simulink model "cpu_sim"  (R2025b)
settings: Solver=VariableStepAuto  StartTime=0.0  StopTime=100  RelTol=1e-3
libraries: simulink x19, hdlsllib x7, embmathops x1
settings Model: Creator=karbi  LastModifiedBy=karbi

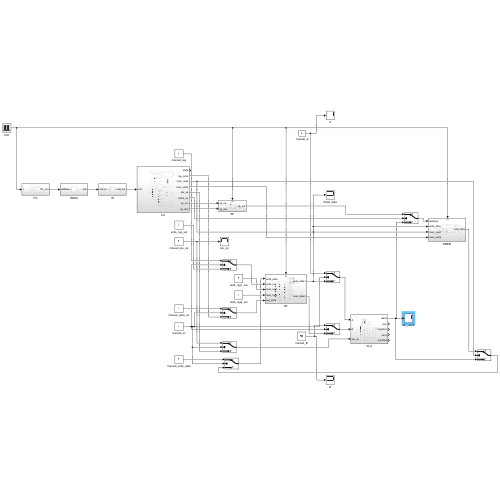
[thumbnail: Simulink's stored preview of the top-level diagram]
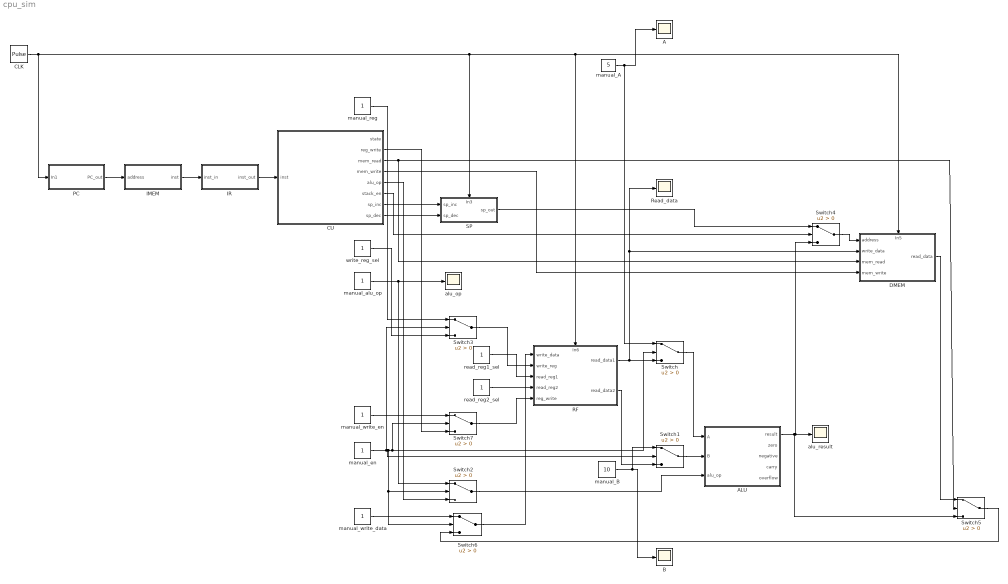
== system cpu_sim ==
  A : Scope
  ALU : Subsystem
  B : Scope
      settings: ActiveDisplayYMinimum=0.50000000000000011  ActiveDisplayYMaximum=5.5
  CLK : DiscretePulseGenerator  PulseType=Time based  Period=10  PulseWidth=5
  CU : Subsystem
  DMEM : Subsystem
      settings: PortSchema="{\"entries\":[{\"content\":{\"sides\":[{\"content\":{\"connectorIds\":[\"In1\",\"In2\",\"In3\",\"In4\"]},\"type\":\"ConnectorPlacement.EquallySpacedRectSide\",\"uuid\":\"c20ba0b8-e86b-4c3c-b1e7-27bfbe6d7ace\"},{\"content\":{\"connectorIds\":[\"Out1\"],\"side\":\"RIGHT\"},\"type\":\"ConnectorPlacement.EquallySpacedRectSide\",\"uuid\":\"6dfc7f35-ab74-4cab-b190-60f3ce7867eb\"},{\"content\":{\"connectorIds\":[\"In5\"],\"side\":\"TOP\"},\"type\":\"ConnectorPlacement.EquallySpacedRectSide\",\"uuid\":\"6a617f88-98bd-4419-a501-824654a091cc\"}]},\"type\":\"ConnectorPlacement.EquallySpacedConnector\",\"uuid\":\"d46b2777-b6fa-41c3-b118-b623252993db\"}],\"packageUris\":[\"http://schema.mathworks.com/mf0/Connector/R2020b\"],\"version\":\"1.0\"}"
  IMEM : Subsystem
  IR : Subsystem
  PC : Subsystem
  RF : Subsystem
      settings: PortSchema="{\"entries\":[{\"content\":{\"sides\":[{\"content\":{\"connectorIds\":[\"In1\",\"In2\",\"In3\",\"In4\",\"In5\"]},\"type\":\"ConnectorPlacement.EquallySpacedRectSide\",\"uuid\":\"b2b0e2f7-f1bc-4913-8ebd-763bbe465d15\"},{\"content\":{\"connectorIds\":[\"Out1\",\"Out2\"],\"side\":\"RIGHT\"},\"type\":\"ConnectorPlacement.EquallySpacedRectSide\",\"uuid\":\"2e2cea93-7dcf-43f8-b2d4-b46fbcb89eb4\"},{\"content\":{\"connectorIds\":[\"In6\"],\"side\":\"TOP\"},\"type\":\"ConnectorPlacement.EquallySpacedRectSide\",\"uuid\":\"73c40681-d123-4d1e-a253-0478733a22e7\"}]},\"type\":\"ConnectorPlacement.EquallySpacedConnector\",\"uuid\":\"66946b18-2392-495c-9280-4c233a61f8fd\"}],\"packageUris\":[\"http://schema.mathworks.com/mf0/Connector/R2020b\"],\"version\":\"1.0\"}"
  Read_data : Scope
      settings: DataLoggingVariableName=ScopeData3
  SP : Subsystem
      settings: PortSchema="{\"entries\":[{\"content\":{\"sides\":[{\"content\":{\"connectorIds\":[\"In1\",\"In2\"]},\"type\":\"ConnectorPlacement.EquallySpacedRectSide\",\"uuid\":\"dbfb5c57-0778-4d2f-89d9-125f1cc5ff40\"},{\"content\":{\"connectorIds\":[\"Out1\"],\"side\":\"RIGHT\"},\"type\":\"ConnectorPlacement.EquallySpacedRectSide\",\"uuid\":\"49ad81b3-cdaa-431a-a3c2-5d84586127d8\"},{\"content\":{\"connectorIds\":[\"In3\"],\"side\":\"TOP\"},\"type\":\"ConnectorPlacement.EquallySpacedRectSide\",\"uuid\":\"61861e8f-55bc-4e95-b317-e383488d79d7\"}]},\"type\":\"ConnectorPlacement.EquallySpacedConnector\",\"uuid\":\"436b8ade-eba4-422b-8f20-150aeb943b61\"}],\"packageUris\":[\"http://schema.mathworks.com/mf0/Connector/R2020b\"],\"version\":\"1.0\"}"
  Switch{,1..7} (8 alike) : Switch  Criteria=u2 > Threshold  SaturateOnIntegerOverflow=off  InputSameDT=off
  alu_op : Scope
      settings: DataLoggingVariableName=ScopeData2
  alu_result : Scope
      settings: ActiveDisplayYMinimum=-0.12200920583340213  ActiveDisplayYMaximum=10.004635007877717  DataLoggingVariableName=ScopeData4
  manual_A : Constant  Value=5  OutDataTypeStr=uint8
  manual_B : Constant  Value=10  OutDataTypeStr=uint8
  manual_alu_op : Constant  OutDataTypeStr=uint8
  manual_en : Constant  OutDataTypeStr=boolean
  manual_reg : Constant  OutDataTypeStr=uint8
  manual_write_data : Constant  OutDataTypeStr=uint8
  manual_write_en : Constant  OutDataTypeStr=boolean
  read_reg1_sel : Constant  OutDataTypeStr=uint8
  read_reg2_sel : Constant  OutDataTypeStr=uint8
  write_reg_sel : Constant  OutDataTypeStr=uint8
  wires:
  CU/4(mem_write) -> DMEM/4(mem_write)
  CU/3(mem_read) -> DMEM/3(mem_read), Switch5/2
  CU/2(reg_write) -> Switch7/3
  CU/6(stack_en) -> Switch4/2
  CLK/1 -> DMEM/5(In5), RF/6(In6), SP/3(In3), PC/1(In1)
  IR/1(inst_out) -> CU/1(inst)
  PC/1(PC_out) -> IMEM/1(address)
  IMEM/1(inst) -> IR/1(inst_in)
  manual_reg/1 -> Switch3/1
  CU/5(alu_op) -> Switch2/3
  CU/7(sp_inc) -> SP/1(sp_inc)
  CU/8(sp_dec) -> SP/2(sp_dec)
  manual_B/1 -> B/1, Switch1/1
  write_reg_sel/1 -> Switch3/3
  manual_alu_op/1 -> Switch2/1, alu_op/1
  manual_write_en/1 -> Switch7/1
  manual_en/1 -> Switch6/2, Switch2/2, Switch7/2, Switch/2, Switch1/2, Switch3/2
  Switch7/1 -> RF/5(reg_write)
  manual_write_data/1 -> Switch6/1
  SP/1(sp_out) -> Switch4/1
  Switch3/1 -> RF/2(write_reg)
  read_reg1_sel/1 -> RF/3(read_reg1)
  manual_A/1 -> Switch/1, A/1
  read_reg2_sel/1 -> RF/4(read_reg2)
  RF/2(read_data2) -> Switch1/3
  Switch2/1 -> ALU/3(alu_op)
  Switch6/1 -> RF/1(write_data)
  RF/1(read_data1) -> Read_data/1, DMEM/2(write_data), Switch/3
  Switch/1 -> ALU/1(A)
  Switch1/1 -> ALU/2(B)
  ALU/1(result) -> alu_result/1, Switch4/3, Switch5/3
  Switch4/1 -> DMEM/1(address)
  DMEM/1(read_data) -> Switch5/1
  Switch5/1 -> Switch6/3

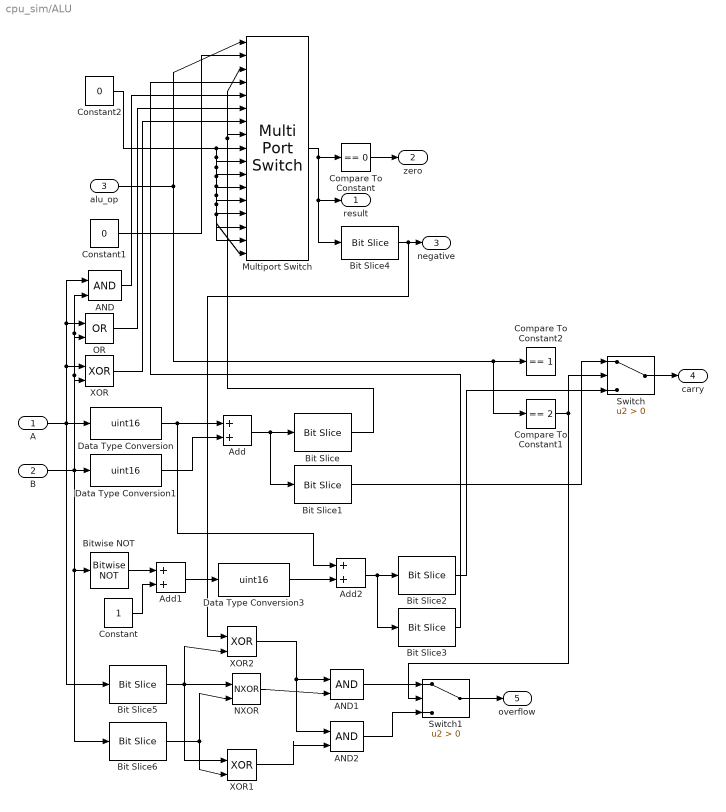
== system cpu_sim/ALU ==
  A : Inport  OutDataTypeStr=uint8
  B : Inport  Port=2  OutDataTypeStr=uint8
  alu_op : Inport  Port=3  OutDataTypeStr=uint8
  AND : Logic  IconShape=distinctive  AllPortsSameDT=off  OutDataTypeStr=boolean
  AND1 : Logic  IconShape=distinctive  AllPortsSameDT=off  OutDataTypeStr=boolean
  AND2 : Logic  IconShape=distinctive  AllPortsSameDT=off  OutDataTypeStr=boolean
  Add : Sum
  Add1 : Sum
  Add2 : Sum  OutDataTypeStr=uint16
  Bit Slice : hdlsllib/Logic and Bit Operations/Bit Slice  lidx=7  ridx=0
  Bit Slice1 : hdlsllib/Logic and Bit Operations/Bit Slice  lidx=8  ridx=8
  Bit Slice2 : hdlsllib/Logic and Bit Operations/Bit Slice  lidx=8  ridx=8
  Bit Slice3 : hdlsllib/Logic and Bit Operations/Bit Slice  lidx=7  ridx=0
  Bit Slice4 : hdlsllib/Logic and Bit Operations/Bit Slice  lidx=7  ridx=7
  Bit Slice5 : hdlsllib/Logic and Bit Operations/Bit Slice  lidx=7  ridx=7
  Bit Slice6 : hdlsllib/Logic and Bit Operations/Bit Slice  lidx=7  ridx=7
  Bitwise NOT : simulink/Logic and Bit Operations/Bitwise Operator  logicop=NOT  UseBitMask=off  BitMask=bin2dec('11011001')  BitMaskRealWorld=Stored Integer
      settings: LibrarySourceBlock=|
      | simulink/Quick Insert/Logic and Bit
      | Operations/Bitwise NOT
  Compare To Constant : simulink/Logic and Bit Operations/Compare To Constant  relop===  const=0  OutDataTypeStr=boolean
  Compare To Constant1 : simulink/Logic and Bit Operations/Compare To Constant  relop===  const=2  OutDataTypeStr=boolean
  Compare To Constant2 : simulink/Logic and Bit Operations/Compare To Constant  relop===  const=1  OutDataTypeStr=boolean
  Constant : Constant
  Constant1 : Constant  Value=0  OutDataTypeStr=uint8
  Constant2 : Constant  Value=0
  Data Type Conversion : DataTypeConversion  OutDataTypeStr=uint16  SaturateOnIntegerOverflow=off  RndMeth=Floor
  Data Type Conversion1 : DataTypeConversion  OutDataTypeStr=uint16  SaturateOnIntegerOverflow=off  RndMeth=Floor
  Data Type Conversion3 : DataTypeConversion  OutDataTypeStr=uint16  SaturateOnIntegerOverflow=off  RndMeth=Floor
  Multiport Switch : MultiPortSwitch  DataPortOrder=Zero-based contiguous  Inputs=16  zeroidx=on  OutDataTypeStr=uint8  SaturateOnIntegerOverflow=off  InputSameDT=off
  NXOR : Logic  Operator=NXOR  IconShape=distinctive  AllPortsSameDT=off  OutDataTypeStr=boolean
  OR : Logic  Operator=OR  IconShape=distinctive  AllPortsSameDT=off  OutDataTypeStr=boolean
  Switch : Switch  Criteria=u2 > Threshold  SaturateOnIntegerOverflow=off  InputSameDT=off
  Switch1 : Switch  Criteria=u2 > Threshold  SaturateOnIntegerOverflow=off  InputSameDT=off
  XOR : Logic  Operator=XOR  IconShape=distinctive  AllPortsSameDT=off  OutDataTypeStr=boolean
  XOR1 : Logic  Operator=XOR  IconShape=distinctive  AllPortsSameDT=off  OutDataTypeStr=boolean
  XOR2 : Logic  Operator=XOR  IconShape=distinctive  AllPortsSameDT=off  OutDataTypeStr=boolean
  result : Outport  OutDataTypeStr=uint8
  zero : Outport  Port=2
  negative : Outport  Port=3
  carry : Outport  Port=4
  overflow : Outport  Port=5
  wires:
  A/1 -> Bit Slice5/1, AND/1, OR/1, XOR/1, Data Type Conversion/1
  B/1 -> XOR/2, OR/2, AND/2, Bit Slice6/1, Bitwise NOT/1, Data Type Conversion1/1
  Data Type Conversion/1 -> Add2/1, Add/1
  Data Type Conversion1/1 -> Add/2
  Add/1 -> Bit Slice1/1, Bit Slice/1
  Bit Slice/1 -> Multiport Switch/8, Multiport Switch/3
  Bit Slice1/1 -> Switch/1
  Bitwise NOT/1 -> Add1/1
  Constant/1 -> Add1/2
  Add1/1 -> Data Type Conversion3/1
  Data Type Conversion3/1 -> Add2/2
  Add2/1 -> Bit Slice3/1, Bit Slice2/1
  Bit Slice2/1 -> Switch/3
  Bit Slice3/1 -> Multiport Switch/4
  alu_op/1 -> Compare To Constant1/1, Compare To Constant2/1, Multiport Switch/1
  Constant1/1 -> Multiport Switch/2
  AND/1 -> Multiport Switch/5
  OR/1 -> Multiport Switch/6
  XOR/1 -> Multiport Switch/7
  Multiport Switch/1 -> Bit Slice4/1, result/1, Compare To Constant/1
  Compare To Constant/1 -> zero/1
  Bit Slice4/1 -> XOR2/1, negative/1
  Compare To Constant1/1 -> Switch1/2, Switch/2
  Switch/1 -> carry/1
  Bit Slice5/1 -> XOR2/2, XOR1/1, NXOR/1
  Bit Slice6/1 -> XOR1/2, NXOR/2
  NXOR/1 -> AND1/2
  XOR2/1 -> AND2/1, AND1/1
  XOR1/1 -> AND2/2
  AND1/1 -> Switch1/1
  AND2/1 -> Switch1/3
  Switch1/1 -> overflow/1
  Constant2/1 -> Multiport Switch/17, Multiport Switch/16, Multiport Switch/15, Multiport Switch/14, Multiport Switch/13, Multiport Switch/12, Multiport Switch/11, Multiport Switch/10, Multiport Switch/9

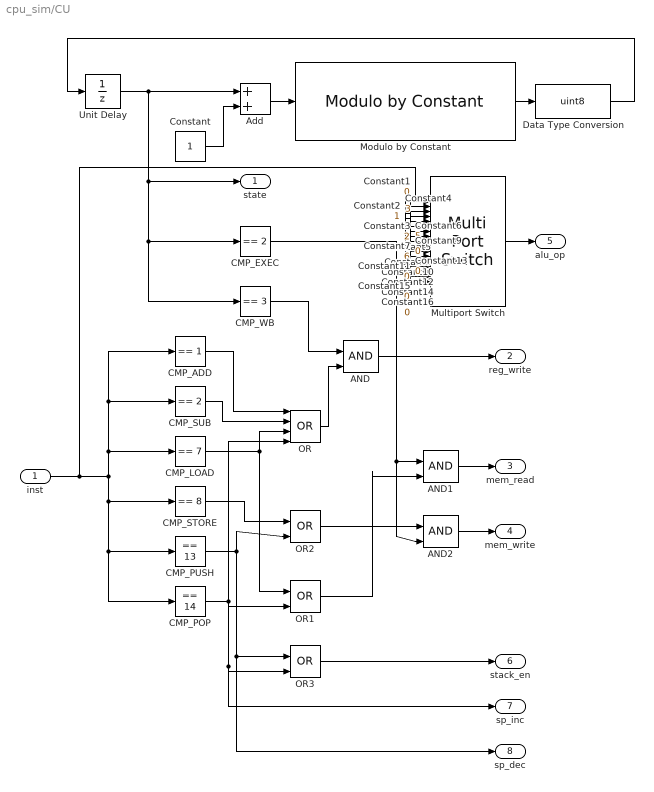
== system cpu_sim/CU ==
  inst : Inport
  AND : Logic  IconShape=distinctive  AllPortsSameDT=off  OutDataTypeStr=boolean
  AND1 : Logic  IconShape=distinctive  AllPortsSameDT=off  OutDataTypeStr=boolean
  AND2 : Logic  IconShape=distinctive  AllPortsSameDT=off  OutDataTypeStr=boolean
  Add : Sum
  CMP_ADD : simulink/Logic and Bit Operations/Compare To Constant  relop===  const=1  OutDataTypeStr=boolean
  CMP_EXEC : simulink/Logic and Bit Operations/Compare To Constant  relop===  const=2  OutDataTypeStr=boolean
  CMP_LOAD : simulink/Logic and Bit Operations/Compare To Constant  relop===  const=7  OutDataTypeStr=boolean
  CMP_POP : simulink/Logic and Bit Operations/Compare To Constant  relop===  const=14  OutDataTypeStr=boolean
  CMP_PUSH : simulink/Logic and Bit Operations/Compare To Constant  relop===  const=13  OutDataTypeStr=boolean
  CMP_STORE : simulink/Logic and Bit Operations/Compare To Constant  relop===  const=8  OutDataTypeStr=boolean
  CMP_SUB : simulink/Logic and Bit Operations/Compare To Constant  relop===  const=2  OutDataTypeStr=boolean
  CMP_WB : simulink/Logic and Bit Operations/Compare To Constant  relop===  const=3  OutDataTypeStr=boolean
  Constant : Constant  OutDataTypeStr=uint8
  Constant{1,8..16} (10 alike) : Constant  Value=0
  Constant2 : Constant
  Constant3 : Constant  Value=2
  Constant4 : Constant  Value=3
  Constant5 : Constant  Value=4
  Constant6 : Constant  Value=5
  Constant7 : Constant  Value=6
  Data Type Conversion : DataTypeConversion  OutDataTypeStr=uint8  SaturateOnIntegerOverflow=off  RndMeth=Floor
  Modulo by Constant : embmathops/Modulo by Constant  Denominator=4  SimulateUsing=Code generation
      settings: LibrarySourceBlock=embeddedMathLib/Modulo by Constant
  Multiport Switch : MultiPortSwitch  DataPortOrder=Zero-based contiguous  Inputs=16  DiagnosticForDefault=None  zeroidx=on  OutDataTypeStr=uint8  SaturateOnIntegerOverflow=off  InputSameDT=off
  OR : Logic  Operator=OR  Inputs=4  IconShape=distinctive  AllPortsSameDT=off  OutDataTypeStr=boolean
  OR1 : Logic  Operator=OR  IconShape=distinctive  AllPortsSameDT=off  OutDataTypeStr=boolean
  OR2 : Logic  Operator=OR  IconShape=distinctive  AllPortsSameDT=off  OutDataTypeStr=boolean
  OR3 : Logic  Operator=OR  IconShape=distinctive  AllPortsSameDT=off  OutDataTypeStr=boolean
  Unit Delay : UnitDelay  SampleTime=-1  HasFrameUpgradeWarning=on
  state : Outport
  reg_write : Outport  Port=2  OutDataTypeStr=boolean
  mem_read : Outport  Port=3  OutDataTypeStr=boolean
  mem_write : Outport  Port=4  OutDataTypeStr=boolean
  alu_op : Outport  Port=5  OutDataTypeStr=uint8
  stack_en : Outport  Port=6  OutDataTypeStr=boolean
  sp_inc : Outport  Port=7  OutDataTypeStr=boolean
  sp_dec : Outport  Port=8  OutDataTypeStr=boolean
  wires:
  Unit Delay/1 -> CMP_WB/1, CMP_EXEC/1, state/1, Add/1
  Constant/1 -> Add/2
  Add/1 -> Modulo by Constant/1
  inst/1 -> Multiport Switch/1, CMP_POP/1, CMP_PUSH/1, CMP_STORE/1, CMP_SUB/1, CMP_ADD/1, CMP_LOAD/1
  CMP_ADD/1 -> OR/1
  CMP_SUB/1 -> OR/2
  CMP_LOAD/1 -> OR1/1, OR/3
  CMP_WB/1 -> AND/1
  OR/1 -> AND/2
  AND/1 -> reg_write/1
  CMP_EXEC/1 -> AND2/2, AND1/1
  CMP_POP/1 -> sp_inc/1, OR3/2, OR/4, OR1/2
  OR1/1 -> AND1/2
  AND1/1 -> mem_read/1
  CMP_STORE/1 -> OR2/1
  CMP_PUSH/1 -> sp_dec/1, OR3/1, OR2/2
  OR2/1 -> AND2/1
  AND2/1 -> mem_write/1
  OR3/1 -> stack_en/1
  Multiport Switch/1 -> alu_op/1
  Constant1/1 -> Multiport Switch/2
  Constant2/1 -> Multiport Switch/3
  Constant3/1 -> Multiport Switch/4
  Constant4/1 -> Multiport Switch/5
  Constant5/1 -> Multiport Switch/6
  Constant6/1 -> Multiport Switch/7
  Constant7/1 -> Multiport Switch/8
  Constant8/1 -> Multiport Switch/9
  Constant9/1 -> Multiport Switch/10
  Constant10/1 -> Multiport Switch/11
  Constant11/1 -> Multiport Switch/12
  Constant12/1 -> Multiport Switch/13
  Constant13/1 -> Multiport Switch/14
  Constant14/1 -> Multiport Switch/15
  Constant15/1 -> Multiport Switch/16
  Constant16/1 -> Multiport Switch/17
  Modulo by Constant/1 -> Data Type Conversion/1
  Data Type Conversion/1 -> Unit Delay/1

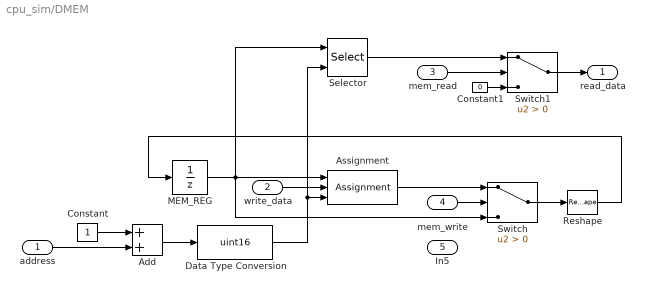
== system cpu_sim/DMEM ==
  address : Inport  OutDataTypeStr=uint8
  write_data : Inport  Port=2  OutDataTypeStr=uint8
  mem_read : Inport  Port=3  OutDataTypeStr=boolean
  mem_write : Inport  Port=4  OutDataTypeStr=boolean
  In5 : Inport  Port=5
  Add : Sum  OutDataTypeStr=uint8
  Assignment : Assignment  IndexMode=Zero-based  DiagnosticForDimensions=Warning  IndexOptions=Index vector (port)  Indices=1  OutputSizes=1
  Constant : Constant  OutDataTypeStr=uint8
  Constant1 : Constant  Value=0  OutDataTypeStr=uint8
  Data Type Conversion : DataTypeConversion  OutDataTypeStr=uint16  SaturateOnIntegerOverflow=off  RndMeth=Floor
  MEM_REG : UnitDelay  InitialCondition=zeros(256,1,'uint8')  SampleTime=-1  HasFrameUpgradeWarning=on
  Reshape : Reshape  OutputDimensionality=Customize  OutputDimensions=[256]
  Selector : Selector  IndexOptions=Index vector (port)  Indices=[1 3]  OutputSizes=1
  Switch : Switch  Criteria=u2 > Threshold  SaturateOnIntegerOverflow=off  InputSameDT=off
  Switch1 : Switch  Criteria=u2 > Threshold  SaturateOnIntegerOverflow=off  InputSameDT=off
  read_data : Outport  OutDataTypeStr=uint8
  wires:
  address/1 -> Add/2
  Add/1 -> Data Type Conversion/1
  Constant/1 -> Add/1
  Data Type Conversion/1 -> Selector/2, Assignment/3
  write_data/1 -> Assignment/2
  Assignment/1 -> Switch/1
  mem_write/1 -> Switch/2
  mem_read/1 -> Switch1/2
  Selector/1 -> Switch1/1
  Constant1/1 -> Switch1/3
  Switch1/1 -> read_data/1
  MEM_REG/1 -> Selector/1, Switch/3, Assignment/1
  Switch/1 -> Reshape/1
  Reshape/1 -> MEM_REG/1

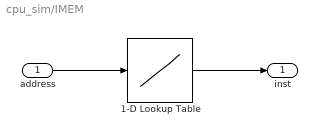
== system cpu_sim/IMEM ==
  address : Inport
  1-D Lookup Table : Lookup_n-D  NumberOfTableDimensions=1  BreakpointsForDimension1=[0:9]  Table=[1 2 3 4 5 6 7 8 9 10]  InterpMethod=Flat  InternalRulePriority=Speed  OutDataTypeStr=uint8  RndMeth=Simplest
  inst : Outport
  wires:
  address/1 -> 1-D Lookup Table/1
  1-D Lookup Table/1 -> inst/1

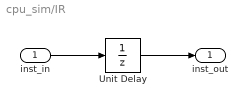
== system cpu_sim/IR ==
  inst_in : Inport
  Unit Delay : UnitDelay  SampleTime=-1  HasFrameUpgradeWarning=on
  inst_out : Outport
  wires:
  inst_in/1 -> Unit Delay/1
  Unit Delay/1 -> inst_out/1

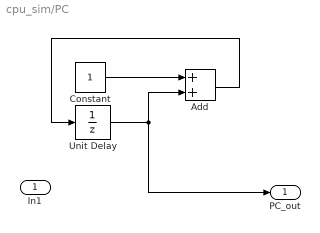
== system cpu_sim/PC ==
  In1 : Inport
  Add : Sum  OutDataTypeStr=uint8
  Constant : Constant
  Unit Delay : UnitDelay  SampleTime=-1  HasFrameUpgradeWarning=on
  PC_out : Outport
  wires:
  Constant/1 -> Add/1
  Unit Delay/1 -> PC_out/1, Add/2
  Add/1 -> Unit Delay/1

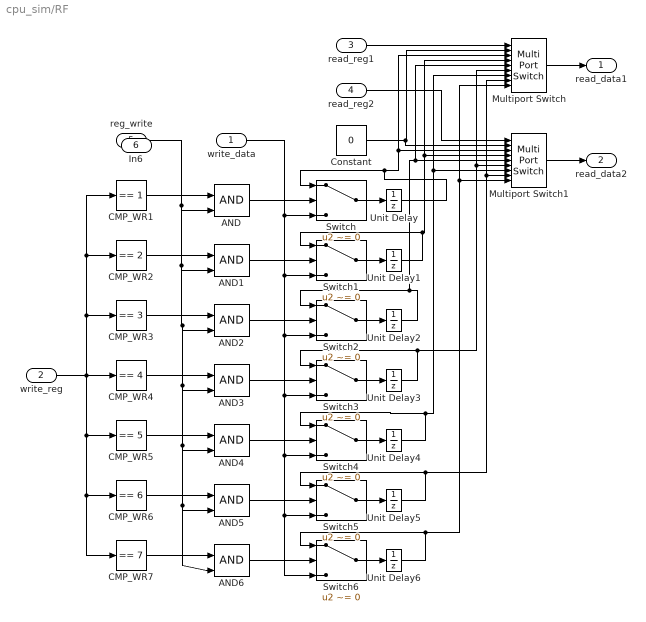
== system cpu_sim/RF ==
  write_data : Inport  OutDataTypeStr=uint8
  write_reg : Inport  Port=2  OutDataTypeStr=uint8
  read_reg1 : Inport  Port=3  OutDataTypeStr=uint8
  read_reg2 : Inport  Port=4  OutDataTypeStr=uint8
  reg_write : Inport  Port=5  OutDataTypeStr=boolean
  In6 : Inport  Port=6
  AND{,1..6} (7 alike) : Logic  IconShape=distinctive  AllPortsSameDT=off  OutDataTypeStr=boolean
  CMP_WR1 : simulink/Logic and Bit Operations/Compare To Constant  relop===  const=1  OutDataTypeStr=boolean
  CMP_WR2 : simulink/Logic and Bit Operations/Compare To Constant  relop===  const=2  OutDataTypeStr=boolean
  "CMP_WR3 " : simulink/Logic and Bit Operations/Compare To Constant  relop===  const=3  OutDataTypeStr=boolean
  CMP_WR4 : simulink/Logic and Bit Operations/Compare To Constant  relop===  const=4  OutDataTypeStr=boolean
  CMP_WR5 : simulink/Logic and Bit Operations/Compare To Constant  relop===  const=5  OutDataTypeStr=boolean
  CMP_WR6 : simulink/Logic and Bit Operations/Compare To Constant  relop===  const=6  OutDataTypeStr=boolean
  CMP_WR7 : simulink/Logic and Bit Operations/Compare To Constant  relop===  const=7  OutDataTypeStr=boolean
  Constant : Constant  Value=0  OutDataTypeStr=uint8
  Multiport Switch : MultiPortSwitch  DataPortOrder=Zero-based contiguous  Inputs=8  zeroidx=on  SaturateOnIntegerOverflow=off  InputSameDT=off
  Multiport Switch1 : MultiPortSwitch  DataPortOrder=Zero-based contiguous  Inputs=8  zeroidx=on  OutDataTypeStr=uint8  SaturateOnIntegerOverflow=off  InputSameDT=off
  Switch{,2..6} (6 alike) : Switch  Criteria=u2 ~= 0  SaturateOnIntegerOverflow=off  InputSameDT=off
  Switch1 : Switch  Criteria=u2 ~= 0  OutDataTypeStr=uint8  SaturateOnIntegerOverflow=off  InputSameDT=off
  Unit Delay{,1..6} (7 alike) : UnitDelay  SampleTime=-1  HasFrameUpgradeWarning=on
  read_data1 : Outport
  read_data2 : Outport  Port=2
  wires:
  write_reg/1 -> CMP_WR7/1, CMP_WR6/1, CMP_WR5/1, CMP_WR1/1, CMP_WR2/1, "CMP_WR3 "/1, CMP_WR4/1
  CMP_WR1/1 -> AND/1
  CMP_WR2/1 -> AND1/1
  "CMP_WR3 "/1 -> AND2/1
  CMP_WR4/1 -> AND3/1
  CMP_WR5/1 -> AND4/1
  CMP_WR6/1 -> AND5/1
  CMP_WR7/1 -> AND6/1
  reg_write/1 -> AND6/2, AND5/2, AND4/2, AND3/2, AND2/2, AND1/2, AND/2
  AND/1 -> Switch/2
  AND1/1 -> Switch1/2
  AND2/1 -> Switch2/2
  AND3/1 -> Switch3/2
  AND4/1 -> Switch4/2
  AND5/1 -> Switch5/2
  AND6/1 -> Switch6/2
  write_data/1 -> Switch6/3, Switch5/3, Switch4/3, Switch3/3, Switch2/3, Switch1/3, Switch/3
  Unit Delay/1 -> Multiport Switch1/3, Multiport Switch/3, Switch/1
  Unit Delay1/1 -> Switch1/1, Multiport Switch1/4, Multiport Switch/4
  Unit Delay2/1 -> Switch2/1, Multiport Switch1/5, Multiport Switch/5
  Unit Delay3/1 -> Switch3/1, Multiport Switch1/6, Multiport Switch/6
  Unit Delay4/1 -> Switch4/1, Multiport Switch1/7, Multiport Switch/7
  Unit Delay5/1 -> Switch5/1, Multiport Switch1/8, Multiport Switch/8
  Unit Delay6/1 -> Switch6/1, Multiport Switch1/9, Multiport Switch/9
  read_reg1/1 -> Multiport Switch/1
  read_reg2/1 -> Multiport Switch1/1
  Constant/1 -> Multiport Switch1/2, Multiport Switch/2
  Multiport Switch1/1 -> read_data2/1
  Multiport Switch/1 -> read_data1/1
  Switch/1 -> Unit Delay/1
  Switch1/1 -> Unit Delay1/1
  Switch2/1 -> Unit Delay2/1
  Switch3/1 -> Unit Delay3/1
  Switch4/1 -> Unit Delay4/1
  Switch5/1 -> Unit Delay5/1
  Switch6/1 -> Unit Delay6/1

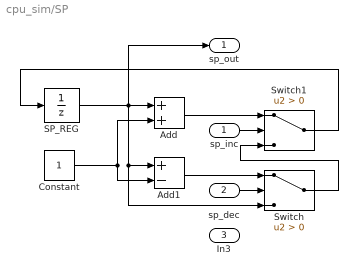
== system cpu_sim/SP ==
  sp_inc : Inport  OutDataTypeStr=boolean
  sp_dec : Inport  Port=2  OutDataTypeStr=boolean
  In3 : Inport  Port=3
  Add : Sum  OutDataTypeStr=uint8
  Add1 : Sum  Inputs=+-  OutDataTypeStr=uint8
  Constant : Constant  OutDataTypeStr=uint8
  SP_REG : UnitDelay  InitialCondition=uint8(255)  SampleTime=-1  HasFrameUpgradeWarning=on
  Switch : Switch  Criteria=u2 > Threshold  SaturateOnIntegerOverflow=off  InputSameDT=off
  Switch1 : Switch  Criteria=u2 > Threshold  SaturateOnIntegerOverflow=off  InputSameDT=off
  sp_out : Outport  OutDataTypeStr=uint8
  wires:
  SP_REG/1 -> sp_out/1, Switch/3, Add1/1, Add/1
  Constant/1 -> Add1/2, Add/2
  Add1/1 -> Switch/1
  sp_dec/1 -> Switch/2
  Add/1 -> Switch1/1
  Switch/1 -> Switch1/3
  sp_inc/1 -> Switch1/2
  Switch1/1 -> SP_REG/1
